simulink library "hydroInversionCoefSensor_cl"  (R2022a)
settings: Solver=VariableStepAuto  StartTime=0.0  StopTime=10.0  RelTol=1e-3
libraries: vrlib x2, vectorNormalizer_ul x2, rotateAboutVec x1, wakeEffect_ul x1
settings Model: Creator=adabney  LastModifiedBy=adabney

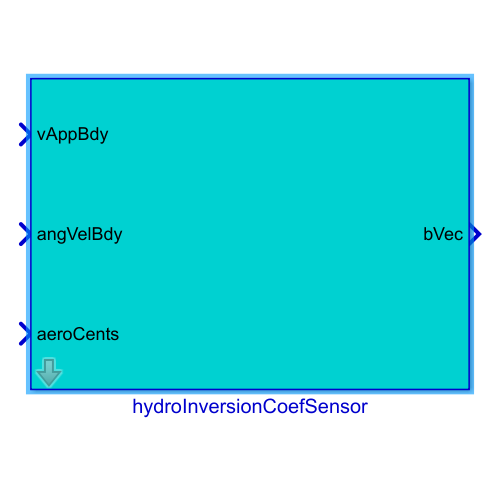
[thumbnail: Simulink's stored preview of the top-level diagram]
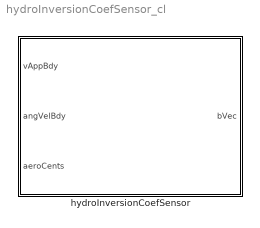
== system hydroInversionCoefSensor_cl ==
  hydroInversionCoefSensor : Subsystem  mask{aeroStruct=0}
      mask prompts: aeroStruct "Aero-surface"

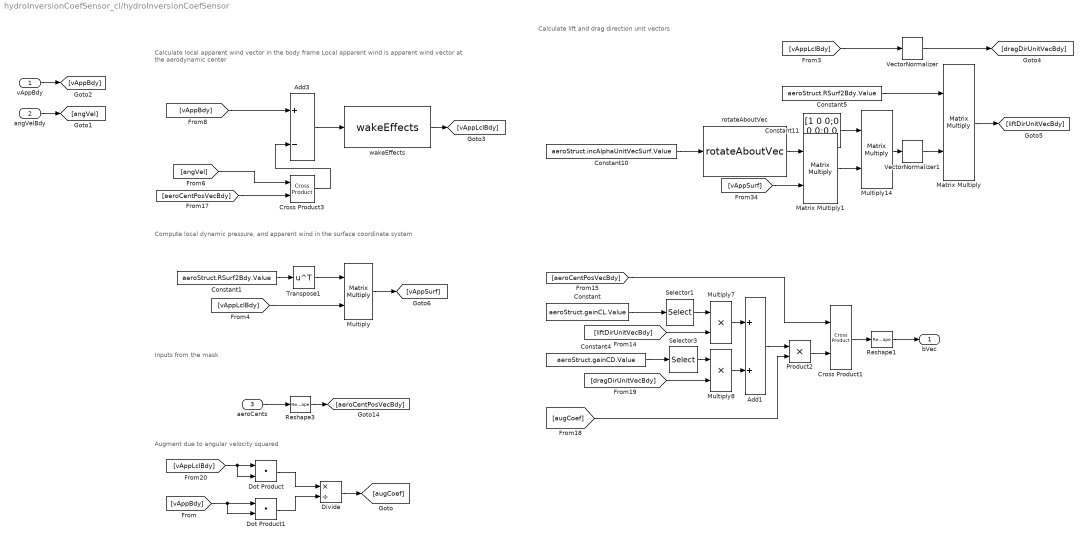
== system hydroInversionCoefSensor_cl/hydroInversionCoefSensor ==
  note: Inputs from the mask
  note: Calculate lift and drag direction unit vectors
  note: Augment due to angular velocity squared
  note: Calculate local apparent wind vector in the body frame
      | Local apparent wind is apparent wind vector at the aerodynamic center
  note: Compute local dynamic pressure,
      | and apparent wind in the surface coordinate system
  vAppBdy : Inport
  angVelBdy : Inport  Port=2
  aeroCents : Inport  Port=3
  Add1 : Sum
  Add3 : Sum  Inputs=+-
  Constant : Constant  Value=aeroStruct.gainCL.Value
  Constant1 : Constant  Value=aeroStruct.RSurf2Bdy.Value
  Constant10 : Constant  Value=aeroStruct.incAlphaUnitVecSurf.Value
  Constant11 : Constant  Value=[1 0 0;0 0 0;0 0 1]
  Constant4 : Constant  Value=aeroStruct.gainCD.Value
  Constant5 : Constant  Value=aeroStruct.RSurf2Bdy.Value
  Cross Product1 : vrlib/Utilities/Cross Product
  Cross Product3 : vrlib/Utilities/Cross Product
  Divide : Product  Inputs=*/
  Dot Product : DotProduct  OutDataTypeStr=Inherit: Inherit via internal rule
  Dot Product1 : DotProduct  OutDataTypeStr=Inherit: Inherit via internal rule
  Matrix Multiply : Product  Multiplication=Matrix(*)
  Matrix Multiply1 : Product  Multiplication=Matrix(*)
  Multiply : Product  Multiplication=Matrix(*)
  Multiply14 : Product  Multiplication=Matrix(*)
  Multiply7 : Product
  Multiply8 : Product
  Product2 : Product
  Reshape1 : Reshape  OutputDimensionality=Column vector (2-D)
  Reshape3 : Reshape  OutputDimensionality=Column vector (2-D)
  Selector1 : Selector  InputPortWidth=3  IndexOptions=Index vector (dialog)  Indices=2  OutputSizes=1
  Selector3 : Selector  InputPortWidth=3  IndexOptions=Index vector (dialog)  Indices=2  OutputSizes=1
  Transpose1 : Math  Operator=transpose  SignedPower=on
  "VectorNormalizer " : vectorNormalizer_ul/VectorNormalizer   SystemSampleTime=-1  VariantActivationTime=update diagram  Latency=0  AutoFrameSizeCalculation=off
  VectorNormalizer1 : vectorNormalizer_ul/VectorNormalizer   SystemSampleTime=-1  VariantActivationTime=update diagram  Latency=0  AutoFrameSizeCalculation=off
  rotateAboutVec : rotateAboutVec/rotateAboutVec  ang=90
  wakeEffects : wakeEffect_ul/wakeEffects  SystemSampleTime=-1  VariantActivationTime=update diagram  Latency=0  AutoFrameSizeCalculation=off
  bVec : Outport  PortDimensions=[3 1]  VectorParamsAs1DForOutWhenUnconnected=off
  wires:
  vAppBdy/1 -> [vAppBdy]
  angVelBdy/1 -> [angVel]
  Selector3/1 -> Multiply8/1
  Product2/1 -> Cross Product1/2
  [augCoef] -> Product2/2
  Add1/1 -> Product2/1
  Matrix Multiply/1 -> [liftDirUnitVecBdy]
  [vAppLclBdy] -> Dot Product/2, Dot Product/1
  [liftDirUnitVecBdy] -> Multiply7/2
  Selector1/1 -> Multiply7/1
  Matrix Multiply1/1 -> Multiply14/2
  Constant5/1 -> Matrix Multiply/1
  Reshape1/1 -> bVec/1
  "VectorNormalizer "/1 -> [dragDirUnitVecBdy]
  VectorNormalizer1/1 -> Matrix Multiply/2
  Constant1/1 -> Transpose1/1
  aeroCents/1 -> Reshape3/1
  Multiply/1 -> [vAppSurf]
  [aeroCentPosVecBdy] -> Cross Product1/1
  Constant11/1 -> Multiply14/1
  [vAppSurf] -> Matrix Multiply1/2
  Multiply14/1 -> VectorNormalizer1/1
  Multiply8/1 -> Add1/2
  Multiply7/1 -> Add1/1
  Add3/1 -> wakeEffects/1
  wakeEffects/1 -> [vAppLclBdy]
  [dragDirUnitVecBdy] -> Multiply8/2
  Dot Product/1 -> Divide/1
  Reshape3/1 -> [aeroCentPosVecBdy]
  [vAppLclBdy] -> Multiply/2
  Constant4/1 -> Selector3/1
  Transpose1/1 -> Multiply/1
  rotateAboutVec/1 -> Matrix Multiply1/1
  Constant/1 -> Selector1/1
  Constant10/1 -> rotateAboutVec/1
  Cross Product1/1 -> Reshape1/1
  [vAppLclBdy] -> "VectorNormalizer "/1
  [angVel] -> Cross Product3/1
  Cross Product3/1 -> Add3/2
  [vAppBdy] -> Add3/1
  [aeroCentPosVecBdy] -> Cross Product3/2
  [vAppBdy] -> Dot Product1/2, Dot Product1/1
  Dot Product1/1 -> Divide/2
  Divide/1 -> [augCoef]
